simulink model "modulation"  (R2021a)
settings: Solver=ode23t  StartTime=0.0  StopTime=1  MaxStep=1e-6  RelTol=1e-3
undefined symbols (not defined in the file): magnitude
libraries: dsparch4 x6, spspowerguiLib x1
settings Model: Creator=DELL  LastModifiedBy=DELL

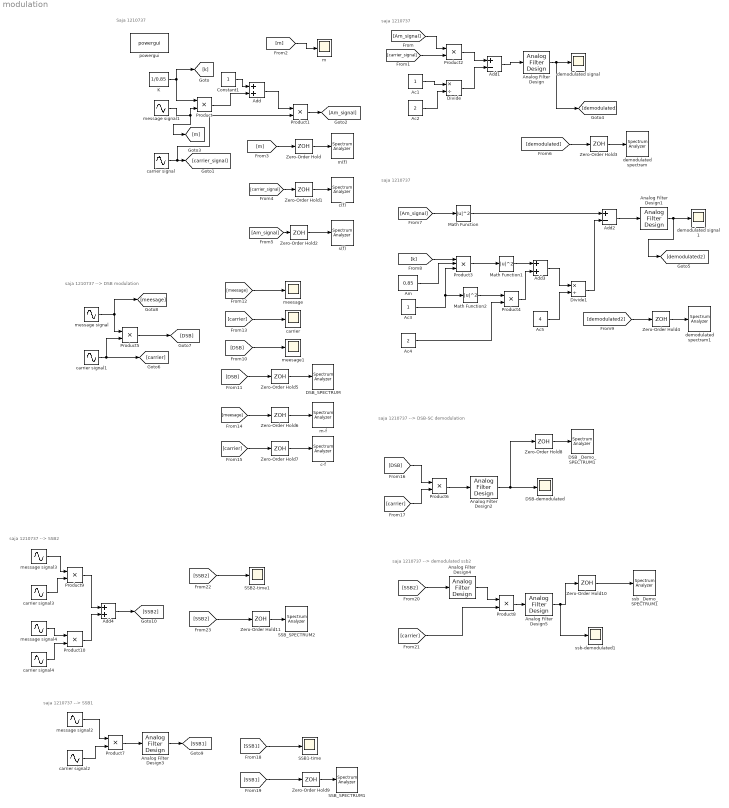
== system modulation ==
  note: saja 1210737 --> SSB2
  note: saja 1210737 --> demodulated ssb2
  note: saja 1210737 --> SSB1
  note: saja 1210737 --> DSB-SC demodulation
  note: saja 1210737 --> DSB modulation
  note: saja 1210737
  note: Saja 1210737
  note: saja 1210737
  Ac1 : Constant
  Ac2 : Constant  Value=2
  Ac3 : Constant
  Ac4 : Constant  Value=2
  Ac5 : Constant  Value=4
  Add : Sum
  Add1 : Sum  Inputs=+-
  Add2 : Sum  Inputs=+-
  Add3 : Sum
  Add4 : Sum
  Am : Constant  Value=0.85
  Analog Filter Design : dsparch4/Analog Filter Design  method=Butterworth  filttype=Lowpass  N=8  Wlo=2*pi*1200  Whi=80  Rp=2  Rs=40
  Analog Filter Design1 : dsparch4/Analog Filter Design  method=Butterworth  filttype=Lowpass  N=8  Wlo=2*pi*1200  Whi=80  Rp=2  Rs=40
  Analog Filter Design2 : dsparch4/Analog Filter Design  method=Butterworth  filttype=Lowpass  N=8  Wlo=2*pi*1200  Whi=2*pi*16e3  Rp=2  Rs=40
  Analog Filter Design3 : dsparch4/Analog Filter Design  method=Butterworth  filttype=Bandpass  N=8  Wlo=2*pi*15e3  Whi=2*pi*17e3  Rp=2  Rs=40
  Analog Filter Design4 : dsparch4/Analog Filter Design  method=Butterworth  filttype=Bandpass  N=8  Wlo=2*pi*15e3  Whi=2*pi*17e3  Rp=2  Rs=40
  Analog Filter Design5 : dsparch4/Analog Filter Design  method=Butterworth  filttype=Lowpass  N=8  Wlo=2*pi*1200  Whi=2*pi*16e3  Rp=2  Rs=40
  Constant1 : Constant
  DSB _Demo_SPECTRUM1 : SpectrumAnalyzer
  DSB-demodulated : Scope
  DSB_SPECTRUM : SpectrumAnalyzer
  Divide : Product  Inputs=*/
  Divide1 : Product  Inputs=*/
  K : Constant  Value=1/0.85
  Math Function : Math  Operator=magnitude^2  SaturateOnIntegerOverflow=on
  Math Function1 : Math  Operator=magnitude^2  SaturateOnIntegerOverflow=on
  Math Function2 : Math  Operator=magnitude^2  SaturateOnIntegerOverflow=on
  Product{,1..2,4..10} (10 alike) : Product
  Product3 : Product  Inputs=3
  SSB1-time : Scope
  SSB2-time1 : Scope
  SSB_SPECTRUM1 : SpectrumAnalyzer
  SSB_SPECTRUM2 : SpectrumAnalyzer
  Zero-Order Hold{,3..4,6,8,10} (6 alike) : ZeroOrderHold  SampleTime=1/(10*1000)
  Zero-Order Hold{1..2,5,7,9,11} (6 alike) : ZeroOrderHold  SampleTime=1/(10*15e3)
  c(f) : SpectrumAnalyzer
  c-f : SpectrumAnalyzer
  carrier : Scope
  carrier signal{,1..4} (5 alike) : Sin  Frequency=2*pi*15e3  Phase=pi/2  SampleTime=0
  "demodulated signal " : Scope
  demodulated signal 1 : Scope
  demodulated spectram : SpectrumAnalyzer
  demodulated spectram1 : SpectrumAnalyzer
  m : Scope
  m(f) : SpectrumAnalyzer
  m-f : SpectrumAnalyzer
  meesage : Scope
  meesage1 : Scope
  message signal{,1..4} (5 alike) : Sin  Amplitude=0.85  Frequency=2*pi*1000  Phase=pi/2  SampleTime=0
  powergui : spspowerguiLib/powergui  Priority=1  SimulationMode=Continuous  SampleTime=50e-6  frequency=60  Iterations=50  frequencyindice=60  Pbase=100e6  ErrMax=1e-4  UnitsV=kV  UnitsW=MW  buscounter=0  FunctionMessages=off  echomessages=off  EnableUseOfTLC=off  CurrentSourceSwitches=off  DisableSnubberDevices=off  DisableRonSwitches=off  DisableVfSwitches=off  DisplayEquations=off  AutomaticDiscreteSolvers=off  SolverType=Tustin/Backward Euler (TBE)  Interpol=off  ExternalGateDelay=off  methode=off  Ts=100  x0status=blocks  SPID=on  SwTol=0  HookPort=off  NonlinearTolerance=1e-4  nMaxIteration=100  ContinueOnMaxIteration=off  RestoreLinks=warning  ResistiveCurrentMeasurement=off  Frange=[0:2:500]  Ylog=off  Xlog=on  ShowGrid=off  save=off  variable=ZData  structure=0  ZoomFFT=off  StartTime=0.0  cycles=1  DisplayStyle=1  fundamental=60  FreqAxis=off  MaxFrequency=1000  frequencyindicesteady=1  RmsSteady=1  display=off
  s(f) : SpectrumAnalyzer
  ssb _Demo_SPECTRUM1 : SpectrumAnalyzer
  ssb-demodulated1 : Scope
  wires:
  Constant1/1 -> Add/1
  Product/1 -> Add/2
  carrier signal/1 -> Product1/2, [carrier_signal]
  Add/1 -> Product1/1
  Product1/1 -> [Am_signal]
  message signal1/1 -> [m], Product/2
  Zero-Order Hold/1 -> m(f)/1
  K/1 -> [k], Product/1
  [m] -> Zero-Order Hold/1
  [carrier_signal] -> Zero-Order Hold1/1
  Zero-Order Hold1/1 -> c(f)/1
  [Am_signal] -> Zero-Order Hold2/1
  Zero-Order Hold2/1 -> s(f)/1
  [demodulated] -> Zero-Order Hold3/1
  [Am_signal] -> Product2/1
  Ac1/1 -> Divide/1
  Analog Filter Design/1 -> [demodulated], "demodulated signal "/1
  Add1/1 -> Analog Filter Design/1
  Product2/1 -> Add1/1
  [carrier_signal] -> Product2/2
  Ac2/1 -> Divide/2
  Divide/1 -> Add1/2
  Zero-Order Hold3/1 -> demodulated spectram/1
  [Am_signal] -> Math Function/1
  Math Function/1 -> Add2/1
  [k] -> Product3/1
  Am/1 -> Product3/2
  Ac3/1 -> Math Function2/1, Product3/3
  Product3/1 -> Math Function1/1
  Math Function1/1 -> Add3/1
  Math Function2/1 -> Product4/1
  Ac4/1 -> Product4/2
  Product4/1 -> Add3/2
  Add3/1 -> Divide1/1
  Ac5/1 -> Divide1/2
  Divide1/1 -> Add2/2
  Add2/1 -> Analog Filter Design1/1
  [m] -> m/1
  Analog Filter Design1/1 -> [demodulated2], demodulated signal 1/1
  [demodulated2] -> Zero-Order Hold4/1
  Zero-Order Hold4/1 -> demodulated spectram1/1
  [DSB] -> Zero-Order Hold5/1
  Zero-Order Hold5/1 -> DSB_SPECTRUM/1
  message signal/1 -> Product5/1, [meesage]
  Product5/1 -> [DSB]
  carrier signal1/1 -> [carrier], Product5/2
  [meesage] -> meesage/1
  [DSB] -> meesage1/1
  [carrier] -> carrier/1
  [meesage] -> Zero-Order Hold6/1
  Zero-Order Hold6/1 -> m-f/1
  [carrier] -> Zero-Order Hold7/1
  Zero-Order Hold7/1 -> c-f/1
  [carrier] -> Product6/2
  Product6/1 -> Analog Filter Design2/1
  Analog Filter Design2/1 -> Zero-Order Hold8/1, DSB-demodulated/1
  [DSB] -> Product6/1
  Zero-Order Hold8/1 -> DSB _Demo_SPECTRUM1/1
  message signal2/1 -> Product7/1
  Zero-Order Hold9/1 -> SSB_SPECTRUM1/1
  [SSB1] -> SSB1-time/1
  [SSB1] -> Zero-Order Hold9/1
  Product7/1 -> Analog Filter Design3/1
  Analog Filter Design3/1 -> [SSB1]
  carrier signal2/1 -> Product7/2
  Analog Filter Design4/1 -> Product8/1
  Product8/1 -> Analog Filter Design5/1
  Zero-Order Hold10/1 -> ssb _Demo_SPECTRUM1/1
  [carrier] -> Product8/2
  [SSB2] -> Analog Filter Design4/1
  Analog Filter Design5/1 -> ssb-demodulated1/1, Zero-Order Hold10/1
  Product9/1 -> Add4/1
  message signal3/1 -> Product9/1
  message signal4/1 -> Product10/1
  Add4/1 -> [SSB2]
  carrier signal4/1 -> Product10/2
  carrier signal3/1 -> Product9/2
  [SSB2] -> Zero-Order Hold11/1
  Zero-Order Hold11/1 -> SSB_SPECTRUM2/1
  [SSB2] -> SSB2-time1/1
  Product10/1 -> Add4/2
